simulink model "controller_geometric"  (R2019b)
settings: Solver=VariableStepAuto  StartTime=0.0  StopTime=10.0  RelTol=1e-3
settings Model: Creator=mummel  LastModifiedBy=mummel

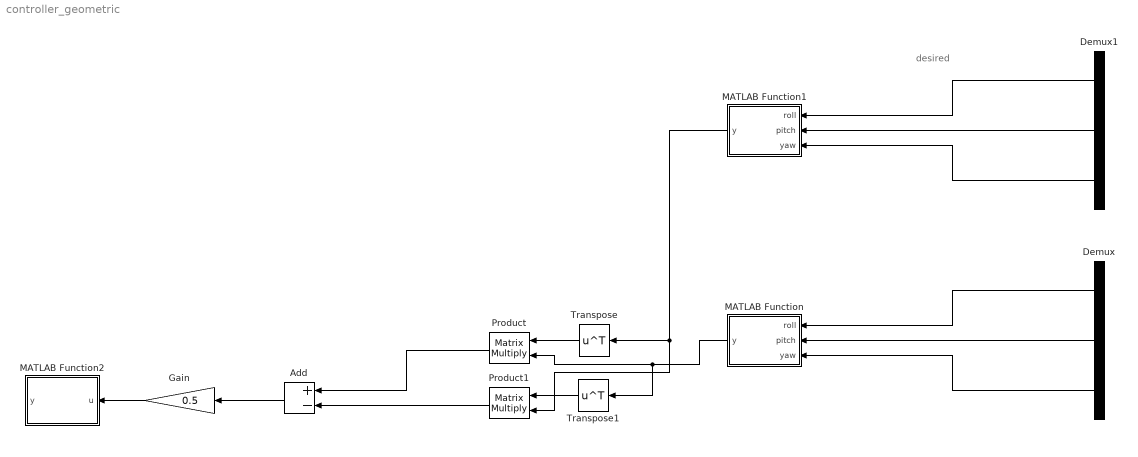
== system controller_geometric ==
  note: desired
  Add : Sum  Inputs=+-
  Demux : Demux  Outputs=3
  Demux1 : Demux  Outputs=3
  Gain : Gain  Gain=0.5
  MATLAB Function : MATLAB Function  TreatAsAtomicUnit=on
  MATLAB Function1 : MATLAB Function  TreatAsAtomicUnit=on
  MATLAB Function2 : MATLAB Function  TreatAsAtomicUnit=on
  Product : Product  Multiplication=Matrix(*)
  Product1 : Product  Multiplication=Matrix(*)
  Transpose : Math  Operator=transpose  SignedPower=off  SaturateOnIntegerOverflow=on
  Transpose1 : Math  Operator=transpose  SignedPower=off  SaturateOnIntegerOverflow=on
  wires:
  Demux/1 -> MATLAB Function/1(roll)
  Demux/2 -> MATLAB Function/2(pitch)
  Demux/3 -> MATLAB Function/3(yaw)
  Demux1/3 -> MATLAB Function1/3(yaw)
  Demux1/1 -> MATLAB Function1/1(roll)
  Demux1/2 -> MATLAB Function1/2(pitch)
  MATLAB Function1/1(y) -> Transpose/1, Product1/2
  Transpose/1 -> Product/1
  MATLAB Function/1(y) -> Transpose1/1, Product/2
  Product/1 -> Add/1
  Product1/1 -> Add/2
  Transpose1/1 -> Product1/1
  Add/1 -> Gain/1
  Gain/1 -> MATLAB Function2/1(u)

== matlab function controller_geometric/MATLAB Function1 ==
  data: roll input; y output; pitch input; yaw input
function y = fcn(roll,pitch,yaw)

y = u;

== matlab function controller_geometric/MATLAB Function ==
  data: roll input; y output; pitch input; yaw input
function y = fcn(roll,pitch,yaw)

y = u;

== matlab function controller_geometric/MATLAB Function2 ==
  data: u input; y output
function y = fcn(u)

y = [u(3,2) u(1,3) u(2,1)];
